simulink model "TestFuncionTransferencia"  (R2023b)
settings: Solver=VariableStepAuto  StartTime=0.0  StopTime=10.0  RelTol=1e-3
settings Model: Creator=Claudia Ada  LastModifiedBy=pablo

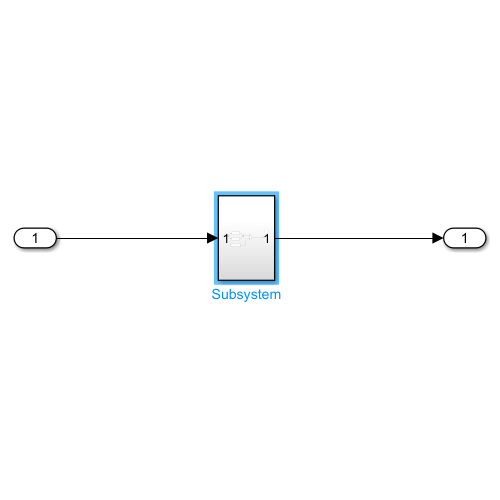
[thumbnail: Simulink's stored preview of the top-level diagram]
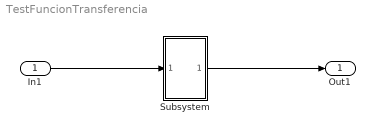
== system TestFuncionTransferencia ==
  In1 : Inport
  Subsystem : Subsystem
  Out1 : Outport
  wires:
  In1/1 -> Subsystem/1(In1)
  Subsystem/1(Out1) -> Out1/1

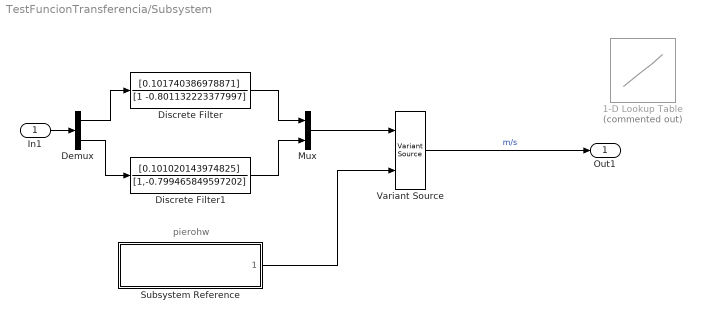
== system TestFuncionTransferencia/Subsystem ==
  note: pierohw
  In1 : Inport
  1-D Lookup Table : Lookup_n-D  Commented=on  NumberOfTableDimensions=1  BreakpointsForDimension1=[-5:5]  Table=tanh([-5:5])  InternalRulePriority=Speed  RndMeth=Simplest
  Demux : Demux  Outputs=2
  Discrete Filter : DiscreteFilter  Numerator=[0.101740386978871]  Denominator=[1 -0.801132223377997]
  Discrete Filter1 : DiscreteFilter  Numerator=[0.101020143974825]  Denominator=[1,-0.799465849597202]
  Mux : Mux  Inputs=2
  Subsystem Reference : Subsystem  ReferencedSubsystem=EncoderBloques
  Variant Source : VariantSource  VariantControlMode=sim codegen switching
  Out1 : Outport
  wires:
  In1/1 -> Demux/1
  Discrete Filter/1 -> Mux/1
  Demux/1 -> Discrete Filter/1
  Discrete Filter1/1 -> Mux/2
  Mux/1 -> Variant Source/1
  Demux/2 -> Discrete Filter1/1
  Subsystem Reference/1 -> Variant Source/2
  Variant Source/1 -> Out1/1  "m/s"
